simulink model "soc_dvbs2_fpga"  (R2025b)
settings: Solver=FixedStepDiscrete  StartTime=0.0  StopTime=0  RelTol=1e-3
InitFcn:
  | soc_dvbs2_init;
values from neighbouring files (symbols this model uses):
  Rsym = 4e6    (= 4000000)    [soc_dvbs2_init.m]
  soc_dvbs2_txPacketBits = [1 1 0 1 0 1 1 1 0 1 1 1 ... (2972 elements, 2972x1)]    [soc_dvbs2_txPacketBits.mat]
  syncWord = (dec2bin(hex2dec('AC')) - '0').'    [soc_dvbs2_init.m]
  txDataOut = txobj(frameBits(:))    [soc_dvbs2_init.m]
  txFiltCoeff = txobj.pTxFilterCoeff    [soc_dvbs2_init.m]
undefined symbols (not defined in the file or in its folder): Add, coefficientsLog, coefficientsSqrt1, coefficientsSqrt2, dataBits, designMultirateFIR, noisePow, NumBits1, NumBits2, seedsURNG1, seedsURNG2, Shift, Slope1, Slope2, soc_dvbs2_designFIRFilter, txDataOutS1, txDataOutS10, txDataOutS12, txDataOutS13, txDataOutS14, txDataOutS15, txDataOutS16, txDataOutS18, txDataOutS19, txDataOutS2, txDataOutS20, txDataOutS21, txDataOutS22, txDataOutS24, txDataOutS25, txDataOutS26, txDataOutS27, txDataOutS3, txDataOutS4, txDataOutS5, txDataOutS6, txDataOutS7, txDataOutS8, txDataOutS9
libraries: simulink x214, hdlsllib x211, dspsigops x22, dsphdlfiltering2 x8, dsphdlsigops2 x5, commseqgen3 x5, dsphdlmathfun2 x3, hwlogicconnlib x2, whdledac x2, commhdlcrc x2, whdlutilities x1, whdlmod x1
(part 1 of 12)
settings Model: DataDictionary=dvbs2hdlReceiverData.sldd  DataTypeOverride=Off  SimulationMode=accelerator  Creator=The MathWorks, Inc.  LastModifiedBy=The MathWorks, Inc.
settings SolverCC: PositivePriorityOrder=on  MaxZcPerStep=1.0
settings DataIOCC: ReturnWorkspaceOutputs=off
settings OptimizationCC: BlockReduction=off  ConditionallyExecuteInputs=off  DefaultParameterBehavior=Inlined  InheritOutputTypeSmallerThanSingle=on  EnhancedBackFolding=on  PassReuseOutputArgsAs=Individual arguments  ZeroExternalMemoryAtStartup=off  ZeroInternalMemoryAtStartup=off  MaxStackSize=64  OptimizeBlockOrder=speed  DifferentSizesBufferReuse=on  OptimizationCustomize=off  EfficientTunableParamExpr=on
settings DebuggingCC: ArtificialAlgebraicLoopMsg=error  SingleTaskRateTransMsg=error  ParameterTunabilityLossMsg=error  UnconnectedInputMsg=warning  UnconnectedOutputMsg=warning  UnconnectedLineMsg=warning  SubsystemReferenceDiagnosticForUnitTest=warning
settings HardwareCC: ProdBitPerPointer=32.0  ProdBitPerSizeT=32.0  ProdBitPerPtrDiffT=32.0  ProdLargestAtomicFloat=None  ProdIntDivRoundTo=Undefined  ProdEndianess=Unspecified  ProdWordSize=32.0  ProdHWDeviceType=ASIC/FPGA->ASIC/FPGA  TargetBitPerLong=64.0  TargetBitPerPointer=64.0  TargetBitPerSizeT=64.0  TargetBitPerPtrDiffT=64.0  TargetLongLongMode=on  TargetIntDivRoundTo=Zero  TargetEndianess=LittleEndian  TargetWordSize=64.0  TargetHWDeviceType=Custom Processor->MATLAB Host Computer  ProdEqTarget=off  HardwareBoardFeatureSet=SoCBlockset
settings ModelReferenceCC: EnableRefExpFcnMdlSchedulingChecks=on
settings RTWCC: SystemTargetFile=ert.tlc  HardwareBoard=Xilinx Zynq UltraScale+ RFSoC ZCU111 Evaluation Kit  TLCOptions="-aInlineSetEventsForThisBaseRateFcn=TLC_FALSE -aSuppressMultiTaskScheduler=TLC_FALSE  -aRateBasedStepFcn=0"  TemplateMakefile=ert_default_tmf  Toolchain=Linaro AArch64 Linux v6.3.1  GPUComputeCapability=3.5  DLArmComputeVersion=19.05  Description=Embedded Coder
settings CodeAppCC: ForceParamTrailComments=on  IgnoreCustomStorageClasses=off  OperatorAnnotations=on  SimulinkDataObjDesc=on  SFDataObjDesc=on  InsertBlockDesc=on

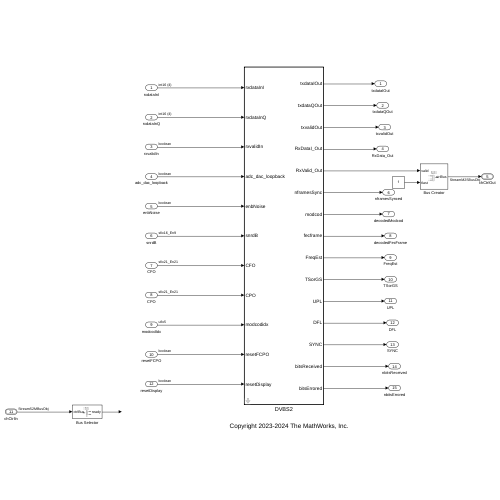
[thumbnail: Simulink's stored preview of the top-level diagram]
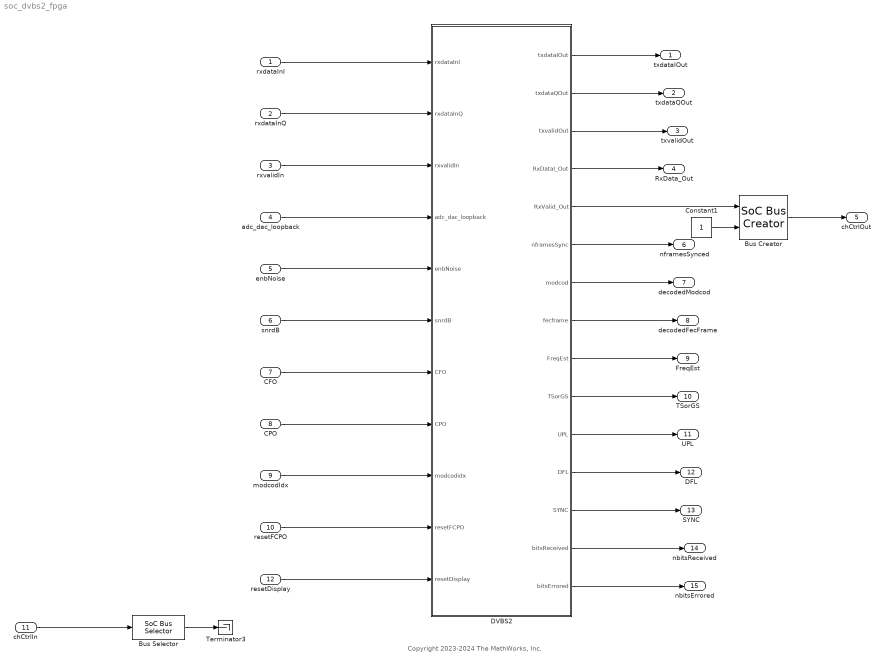
== system soc_dvbs2_fpga ==
  note: Copyright 2023-2024 The MathWorks, Inc.
  rxdataInI : Inport  OutDataTypeStr=int16  PortDimensions=4  LockScale=on
  rxdataInQ : Inport  Port=2  OutDataTypeStr=int16  PortDimensions=4  LockScale=on
  rxvalidIn : Inport  Port=3  OutDataTypeStr=boolean  LockScale=on
  adc_dac_loopback : Inport  Port=4  OutDataTypeStr=boolean  LockScale=on
  enbNoise : Inport  Port=5  OutDataTypeStr=boolean
  snrdB : Inport  Port=6  OutDataTypeStr=fixdt(1,16,9)
  CFO : Inport  Port=7  OutDataTypeStr=fixdt(1,21,21)
  CPO : Inport  Port=8  OutDataTypeStr=fixdt(1,21,21)
  modcodIdx : Inport  Port=9  OutDataTypeStr=fixdt(0,5,0)
  resetFCPO : Inport  Port=10  OutDataTypeStr=boolean
  chCtrlIn : Inport  Port=11  OutDataTypeStr=Bus: StreamS2MBusObj  BusOutputAsStruct=on
  resetDisplay : Inport  Port=12  OutDataTypeStr=boolean
  Bus Creator : hwlogicconnlib/SoC Bus Creator  Protocol=Data stream  ctrltype=Valid
  Bus Selector : hwlogicconnlib/SoC Bus Selector  Protocol=Data stream  ctrltype=Ready
  Constant1 : Constant  OutDataTypeStr=boolean  SampleTime=-1
  DVBS2 : Subsystem  TreatAsAtomicUnit=on
      mask init:
      | coe = designMultirateFIR(1,8); %#ok<NASGU> 
      | interp_coeff = designMultirateFIR(8,1,16); %#ok<NASGU> 
      | Simulink.suppressDiagnostic(gcb, 'SimulinkFixedPoint:util:fxpParameterPrecisionLoss');
  Terminator3 : Terminator
  txdataIOut : Outport
  txdataQOut : Outport  Port=2
  txvalidOut : Outport  Port=3
  RxData_Out : Outport  Port=4
  chCtrlOut : Outport  Port=5  OutDataTypeStr=Bus: StreamM2SBusObj  VectorParamsAs1DForOutWhenUnconnected=off  BusOutputAsStruct=on
  nframesSynced : Outport  Port=6
  decodedModcod : Outport  Port=7
  decodedFecFrame : Outport  Port=8
  FreqEst : Outport  Port=9
  TSorGS : Outport  Port=10
  UPL : Outport  Port=11
  DFL : Outport  Port=12
  SYNC : Outport  Port=13
  nbitsReceived : Outport  Port=14
  nbitsErrored : Outport  Port=15
  wires:
  rxdataInI/1 -> DVBS2/1(rxdataInI)
  rxdataInQ/1 -> DVBS2/2(rxdataInQ)
  rxvalidIn/1 -> DVBS2/3(rxvalidIn)
  adc_dac_loopback/1 -> DVBS2/4(adc_dac_loopback)
  snrdB/1 -> DVBS2/6(snrdB)
  CPO/1 -> DVBS2/8(CPO)
  modcodIdx/1 -> DVBS2/9(modcodidx)
  enbNoise/1 -> DVBS2/5(enbNoise)
  DVBS2/3(txvalidOut) -> txvalidOut/1
  DVBS2/6(nframesSync) -> nframesSynced/1
  DVBS2/7(modcod) -> decodedModcod/1
  DVBS2/8(fecframe) -> decodedFecFrame/1
  DVBS2/9(FreqEst) -> FreqEst/1
  resetFCPO/1 -> DVBS2/10(resetFCPO)
  DVBS2/4(RxDataI_Out) -> RxData_Out/1
  Bus Creator/1 -> chCtrlOut/1
  DVBS2/5(RxValid_Out) -> Bus Creator/1
  Constant1/1 -> Bus Creator/2
  chCtrlIn/1 -> Bus Selector/1
  Bus Selector/1 -> Terminator3/1
  CFO/1 -> DVBS2/7(CFO)
  DVBS2/1(txdataIOut) -> txdataIOut/1
  DVBS2/2(txdataQOut) -> txdataQOut/1
  DVBS2/11(UPL) -> UPL/1
  DVBS2/13(SYNC) -> SYNC/1
  DVBS2/10(TSorGS) -> TSorGS/1
  DVBS2/12(DFL) -> DFL/1
  DVBS2/14(bitsReceived) -> nbitsReceived/1
  DVBS2/15(bitsErrored) -> nbitsErrored/1
  resetDisplay/1 -> DVBS2/11(resetDisplay)

== system soc_dvbs2_fpga/DVBS2 ==
  rxdataInI : Inport
  rxdataInQ : Inport  Port=2
  rxvalidIn : Inport  Port=3
  adc_dac_loopback : Inport  Port=4
  enbNoise : Inport  Port=5
  snrdB : Inport  Port=6
  CFO : Inport  Port=7
  CPO : Inport  Port=8
  modcodidx : Inport  Port=9
  resetFCPO : Inport  Port=10
  resetDisplay : Inport  Port=11
  BER : Subsystem
  Bit Shift : hdlsllib/Logic and Bit Operations/Bit Shift  mode=Shift Left Logical  N=2
  Bit Shift1 : hdlsllib/Logic and Bit Operations/Bit Shift  mode=Shift Left Logical  N=2
  Concatention : Subsystem  TreatAsAtomicUnit=on
  DVBS2 TxRx : Subsystem
  Downsample{,1..6} (7 alike) : DownSample  N=8  RateOptions=Allow multirate processing
  Repeat{,1..2,4} (4 alike) : dspsigops/Repeat  FactorSource=Dialog parameter  N=32  Nmax=16  RateOptions=Allow multirate processing  ic=0  mode=Unused parameter value
  Upsample : dspsigops/Upsample  FactorSource=Dialog parameter  N=32  Nmax=16  phase=0  RateOptions=Allow multirate processing  ic=0  mode=Unused parameter value
  Upsample1 : dspsigops/Upsample  FactorSource=Dialog parameter  N=32  Nmax=16  phase=0  RateOptions=Allow multirate processing  ic=0  mode=Unused parameter value
  Vector Decimation : Subsystem
  Vector Interpolation : Subsystem
  txdataIOut : Outport
  txdataQOut : Outport  Port=2
  txvalidOut : Outport  Port=3
  RxDataI_Out : Outport  Port=4
  RxValid_Out : Outport  Port=5
  nframesSync : Outport  Port=6
  modcod : Outport  Port=7
  fecframe : Outport  Port=8
  FreqEst : Outport  Port=9
  TSorGS : Outport  Port=10
  UPL : Outport  Port=11
  DFL : Outport  Port=12
  SYNC : Outport  Port=13
  bitsReceived : Outport  Port=14
  bitsErrored : Outport  Port=15
  wires:
  adc_dac_loopback/1 -> Downsample/1
  CFO/1 -> Downsample3/1
  snrdB/1 -> Downsample2/1
  CPO/1 -> Downsample4/1
  resetFCPO/1 -> Downsample6/1
  modcodidx/1 -> Downsample5/1
  enbNoise/1 -> Downsample1/1
  DVBS2 TxRx/1(txDataI_Out) -> Vector Interpolation/1(dataI_in)
  DVBS2 TxRx/2(txDataQ_Out) -> Vector Interpolation/2(dataQ_in)
  DVBS2 TxRx/3(txValid_Out) -> Vector Interpolation/3(valid)
  Concatention/1(dataOut) -> RxDataI_Out/1
  Repeat/1 -> nframesSync/1
  Repeat1/1 -> modcod/1
  Repeat2/1 -> fecframe/1
  Repeat4/1 -> FreqEst/1
  Upsample/1 -> Concatention/1(dataIn)
  Upsample1/1 -> RxValid_Out/1
  Vector Decimation/1(dataIOut) -> DVBS2 TxRx/1(rxExtdataI_In)
  Vector Decimation/2(dataQOut) -> DVBS2 TxRx/2(rxExtdataQ_In)
  Vector Decimation/3(validOut) -> DVBS2 TxRx/3(rxExtValid_In)
  rxdataInI/1 -> Vector Decimation/1(dataI_in)
  rxvalidIn/1 -> Vector Decimation/3(validIn)
  Vector Interpolation/1(txIData) -> Bit Shift/1
  Vector Interpolation/2(txQData) -> Bit Shift1/1
  Vector Interpolation/3(txValid) -> txvalidOut/1
  rxdataInQ/1 -> Vector Decimation/2(dataQ_in)
  Bit Shift/1 -> txdataIOut/1
  Bit Shift1/1 -> txdataQOut/1
  DVBS2 TxRx/4(constlOut) -> Upsample/1
  DVBS2 TxRx/5(constlValid) -> Upsample1/1
  DVBS2 TxRx/6(nframesSync) -> Repeat/1
  DVBS2 TxRx/7(modcod) -> Repeat1/1
  DVBS2 TxRx/8(fecFrame) -> Repeat2/1
  DVBS2 TxRx/9(FreqEst) -> Repeat4/1
  DVBS2 TxRx/12(DFL) -> DFL/1
  DVBS2 TxRx/11(UPL) -> UPL/1
  DVBS2 TxRx/10(TsorGS) -> TSorGS/1
  DVBS2 TxRx/13(SYNC) -> SYNC/1
  DVBS2 TxRx/14(bitsOut) -> BER/1(userBits)
  DVBS2 TxRx/15(startOut) -> BER/2(srt)
  DVBS2 TxRx/16(endOut) -> BER/3(end)
  DVBS2 TxRx/17(validOut) -> BER/4(userBitsValid)
  DVBS2 TxRx/18(invalidPkt) -> BER/5(invalid)
  BER/1(bitCount) -> bitsReceived/1
  BER/2(bitErrors) -> bitsErrored/1
  resetDisplay/1 -> BER/6(resetcounter)
  Downsample/1 -> DVBS2 TxRx/4(adc_dac_loopback)
  Downsample1/1 -> DVBS2 TxRx/5(enNoise)
  Downsample2/1 -> DVBS2 TxRx/6(snrdB)
  Downsample3/1 -> DVBS2 TxRx/7(CFO)
  Downsample4/1 -> DVBS2 TxRx/8(CPO)
  Downsample5/1 -> DVBS2 TxRx/9(modcodidx)
  Downsample6/1 -> DVBS2 TxRx/10(rstFCPO)

== system soc_dvbs2_fpga/DVBS2/BER ==
  userBits : Inport
  srt : Inport  Port=2
  end : Inport  Port=3
  userBitsValid : Inport  Port=4
  invalid : Inport  Port=5
  resetcounter : Inport  Port=6
  Compare To Constant : simulink/Logic and Bit Operations/Compare To Constant  relop===  const=0  OutDataTypeStr=boolean
  Data Type Conversion1 : DataTypeConversion  OutDataTypeStr=boolean  SaturateOnIntegerOverflow=off  RndMeth=Floor
  Delay : Delay  DelayLength=1
  Delay1 : Delay  DelayLength=1
  Delay4 : Delay  DelayLength=1550
  Delay5 : Delay  DelayLength=1550
  Delay6 : Delay  DelayLength=1550
  HDL Counter : hdlsllib/Sources/HDL Counter  CountType=Free running  CountInit=0  CountStep=1  CountMax=25  CountFromType=Initial value  CountFrom=0  CountResetPort=on  CountLoadPort=off  CountEnbPort=on  CountDirPort=off  CountHitOutputPort=off  CountDataType=Unsigned  CountWordLen=32  CountFracLen=0  CountSampTime=1
  HDL Counter1 : hdlsllib/Sources/HDL Counter  CountType=Free running  CountInit=0  CountStep=1  CountMax=25  CountFromType=Initial value  CountFrom=0  CountResetPort=on  CountLoadPort=off  CountEnbPort=on  CountDirPort=off  CountHitOutputPort=off  CountDataType=Unsigned  CountWordLen=32  CountFracLen=0  CountSampTime=1
  Logical Operator : Logic  AllPortsSameDT=off  OutDataTypeStr=boolean
  Logical Operator1 : Logic  Operator=OR  AllPortsSameDT=off  OutDataTypeStr=boolean
  Logical Operator2 : Logic  Operator=NOT  AllPortsSameDT=off  OutDataTypeStr=boolean
  Logical Operator3 : Logic  AllPortsSameDT=off  OutDataTypeStr=boolean
  Relational Operator : RelationalOperator  Operator=~=  OutDataTypeStr=boolean  InputSameDT=off
  Send Payload Data : Subsystem  TreatAsAtomicUnit=on
  Unit Delay Enabled Synchronous : hdlsllib/Discrete/Unit Delay Enabled Synchronous  InitialCondition=0.0  SampleTime=-1
  Unit Delay Enabled Synchronous1 : hdlsllib/Discrete/Unit Delay Enabled Synchronous  InitialCondition=0.0  SampleTime=-1
  bitCount : Outport  VectorParamsAs1DForOutWhenUnconnected=off
  bitErrors : Outport  Port=2  VectorParamsAs1DForOutWhenUnconnected=off
  wires:
  Delay/1 -> Relational Operator/1
  Logical Operator3/1 -> Send Payload Data/2(nxtBit), HDL Counter1/2, Logical Operator/1
  Send Payload Data/1(dataIn) -> Data Type Conversion1/1
  Data Type Conversion1/1 -> Relational Operator/2
  Relational Operator/1 -> Logical Operator/2
  Logical Operator/1 -> HDL Counter/2
  HDL Counter1/1 -> Compare To Constant/1, bitCount/1
  HDL Counter/1 -> bitErrors/1
  srt/1 -> Delay6/1
  Compare To Constant/1 -> Logical Operator1/1
  Logical Operator1/1 -> HDL Counter/1
  resetcounter/1 -> Logical Operator1/2, HDL Counter1/1
  userBits/1 -> Delay5/1
  userBitsValid/1 -> Delay4/1
  invalid/1 -> Unit Delay Enabled Synchronous/1
  end/1 -> Unit Delay Enabled Synchronous/2
  Delay4/1 -> Delay1/1
  Delay5/1 -> Delay/1
  Delay6/1 -> Unit Delay Enabled Synchronous1/2, Send Payload Data/1(rst)
  Unit Delay Enabled Synchronous/1 -> Logical Operator2/1
  Logical Operator2/1 -> Unit Delay Enabled Synchronous1/1
  Delay1/1 -> Logical Operator3/2
  Unit Delay Enabled Synchronous1/1 -> Logical Operator3/1

== system soc_dvbs2_fpga/DVBS2/Concatention ==
  dataIn : Inport
  Bit Concat : hdlsllib/Logic and Bit Operations/Bit Concat  numInputs=2
  Complex to Real-Imag1 : ComplexToRealImag
  Data Type Conversion : DataTypeConversion  OutDataTypeStr=fixdt(1,16,12)  SaturateOnIntegerOverflow=off  RndMeth=Floor
  Data Type Conversion1 : DataTypeConversion  OutDataTypeStr=int16  ConvertRealWorld=Stored Integer (SI)  SaturateOnIntegerOverflow=off  RndMeth=Floor
  dataOut : Outport
  wires:
  Bit Concat/1 -> dataOut/1
  dataIn/1 -> Data Type Conversion/1
  Complex to Real-Imag1/1 -> Bit Concat/1
  Complex to Real-Imag1/2 -> Bit Concat/2
  Data Type Conversion/1 -> Data Type Conversion1/1
  Data Type Conversion1/1 -> Complex to Real-Imag1/1

== system soc_dvbs2_fpga/DVBS2/DVBS2 TxRx ==
  rxExtdataI_In : Inport
  rxExtdataQ_In : Inport  Port=2
  rxExtValid_In : Inport  Port=3
  adc_dac_loopback : Inport  Port=4
  enNoise : Inport  Port=5
  snrdB : Inport  Port=6
  CFO : Inport  Port=7
  CPO : Inport  Port=8
  modcodidx : Inport  Port=9
  rstFCPO : Inport  Port=10
  Bus Selector : BusSelector  OutputSignals=TSorGS,UPL,DFL,SYNC
  Channel : Subsystem
  Complex to Real-Imag : ComplexToRealImag
  DVB-S2 HDL Receiver : Subsystem
  Digital Automatic Gain Control : Subsystem  mask{desiredOutputPower=0.25, stepSize=(5e-4)}
      mask prompts: desiredOutputPower "Desired output power:"; stepSize "Adaptation step size:"
      mask init:
      | validateattributes(desiredOutputPower,{'double'},{'scalar','real','>=',0.125,'<=',2},'','desired output power');
      |    validateattributes(stepSize,{'double'},{'scalar','real','>=',0.5e-4,'<=',15e-4},'','step size');
      |    if desiredOutputPower > 1
      |        slopeAdj = 2^nextpow2(desiredOutputPower); %#ok<NASGU> 
      |    else
      |        slopeAdj = 1; %#ok<NASGU> 
      |    end
      mask DialogControl DescGroupVar Prompt: Digital Automatic Gain Control
      mask DialogControl DescTextVar Prompt: This block uses feedback loop based gain correction that adjusts adaptively to set the output signal level to reference level.
      mask Display:
      | dispstr1 = 'Digital AGC';
      | disp(dispstr1);
  Downsample7 : DownSample  N=4  RateOptions=Allow multirate processing
  LUT Based Tx : Subsystem
  Prepare Inputs : Subsystem
  Prepare Outputs : Subsystem
  Real-Imag to Complex : RealImagToComplex
  Switch : Switch  Criteria=u2 ~= 0  SaturateOnIntegerOverflow=off  InputSameDT=off
  Switch1 : Switch  Criteria=u2 ~= 0  SaturateOnIntegerOverflow=off  InputSameDT=off
  Terminator : Terminator
  Terminator1 : Terminator
  txDataI_Out : Outport
  txDataQ_Out : Outport  Port=2
  txValid_Out : Outport  Port=3
  constlOut : Outport  Port=4
  constlValid : Outport  Port=5
  nframesSync : Outport  Port=6
  modcod : Outport  Port=7
  fecFrame : Outport  Port=8
  FreqEst : Outport  Port=9
  TsorGS : Outport  Port=10
  UPL : Outport  Port=11
  DFL : Outport  Port=12
  SYNC : Outport  Port=13
  bitsOut : Outport  Port=14
  startOut : Outport  Port=15
  endOut : Outport  Port=16
  validOut : Outport  Port=17
  invalidPkt : Outport  Port=18
  wires:
  Switch/1 -> Digital Automatic Gain Control/1(dataIn)
  Switch1/1 -> Digital Automatic Gain Control/2(validIn)
  Digital Automatic Gain Control/1(dataOut) -> DVB-S2 HDL Receiver/1(dataIn)
  Digital Automatic Gain Control/2(validOut) -> DVB-S2 HDL Receiver/2(validIn)
  LUT Based Tx/2(txValidOut) -> Prepare Outputs/2(txvalid), Channel/2(txValidOut)
  adc_dac_loopback/1 -> Switch/2, Switch1/2
  CFO/1 -> Channel/5(CFO)
  snrdB/1 -> Channel/3(snrdB)
  CPO/1 -> Channel/6(CPO)
  rstFCPO/1 -> DVB-S2 HDL Receiver/3(rstFCPO)
  enNoise/1 -> Channel/4(enNoise)
  rxExtdataI_In/1 -> Real-Imag to Complex/1
  rxExtdataQ_In/1 -> Real-Imag to Complex/2
  Real-Imag to Complex/1 -> Prepare Inputs/1(rxData)
  rxExtValid_In/1 -> Prepare Inputs/2(rxValid)
  Prepare Inputs/2(rxValidOut) -> Switch1/1
  Complex to Real-Imag/1 -> txDataI_Out/1
  Complex to Real-Imag/2 -> txDataQ_Out/1
  Prepare Inputs/1(rxDataOut) -> Switch/1
  Channel/2(validOut) -> Switch1/3
  Channel/1(dataOut) -> Switch/3
  modcodidx/1 -> Downsample7/1
  Downsample7/1 -> LUT Based Tx/1(modcodidx)
  DVB-S2 HDL Receiver/1(syncSymb) -> constlOut/1
  DVB-S2 HDL Receiver/2(syncSymbValid) -> constlValid/1
  DVB-S2 HDL Receiver/3(numSynced) -> nframesSync/1
  DVB-S2 HDL Receiver/4(MODCOD) -> modcod/1
  DVB-S2 HDL Receiver/5(fecFrame) -> fecFrame/1
  DVB-S2 HDL Receiver/6(fineFreqEst) -> FreqEst/1
  DVB-S2 HDL Receiver/7(bitsOut) -> bitsOut/1
  DVB-S2 HDL Receiver/11(errorOut) -> Terminator/1
  DVB-S2 HDL Receiver/8(startOut) -> startOut/1
  DVB-S2 HDL Receiver/9(endOut) -> endOut/1
  DVB-S2 HDL Receiver/10(validOut) -> validOut/1
  DVB-S2 HDL Receiver/12(invalidPkt) -> invalidPkt/1
  DVB-S2 HDL Receiver/13(BBHeaderCRCInfo) -> Terminator1/1
  DVB-S2 HDL Receiver/14(BBheaderParams) -> Bus Selector/1
  Bus Selector/1 -> TsorGS/1  "<TSorGS>"
  Bus Selector/2 -> UPL/1  "<UPL>"
  Bus Selector/3 -> DFL/1  "<DFL>"
  Bus Selector/4 -> SYNC/1  "<SYNC>"
  LUT Based Tx/1(txDataOut) -> Channel/1(txDataOut), Prepare Outputs/1(txData)
  Prepare Outputs/2(txValidOut) -> txValid_Out/1
  Prepare Outputs/1(txDataOut) -> Complex to Real-Imag/1

== system soc_dvbs2_fpga/DVBS2/Vector Decimation ==
  dataI_in : Inport
  dataQ_in : Inport  Port=2
  validIn : Inport  Port=3  PortDimensions=1
  Bit Shift : hdlsllib/Logic and Bit Operations/Bit Shift  mode=Shift Left Logical  N=4
  Complex to Real-Imag : ComplexToRealImag
  Vector Decimation : Subsystem
  dataIOut : Outport
  dataQOut : Outport  Port=2
  validOut : Outport  Port=3
  wires:
  Complex to Real-Imag/2 -> dataQOut/1
  Complex to Real-Imag/1 -> dataIOut/1
  validIn/1 -> Vector Decimation/3(vin)
  Vector Decimation/2(vout) -> validOut/1
  dataQ_in/1 -> Vector Decimation/2(din_img)
  Vector Decimation/1(dout) -> Bit Shift/1
  dataI_in/1 -> Vector Decimation/1(din_real)
  Bit Shift/1 -> Complex to Real-Imag/1

== system soc_dvbs2_fpga/DVBS2/Vector Interpolation ==
  dataI_in : Inport
  dataQ_in : Inport  Port=2
  valid : Inport  Port=3
  Complex to Real-Imag : ComplexToRealImag
  Data Type Conversion3 : DataTypeConversion  OutDataTypeStr=int16  SaturateOnIntegerOverflow=off  RndMeth=Floor
  Data Type Conversion4 : DataTypeConversion  OutDataTypeStr=int16  SaturateOnIntegerOverflow=off  RndMeth=Floor
  Extract Bits1 : simulink/Logic and Bit Operations/Extract Bits  bitsToExtract=Range starting with most significant bit  numBits=12  bitIdxRange=[0 7]  outScalingMode=Treat bit field as an integer
  Extract Bits2 : simulink/Logic and Bit Operations/Extract Bits  bitsToExtract=Range starting with most significant bit  numBits=12  bitIdxRange=[0 7]  outScalingMode=Treat bit field as an integer
  FIR Interpolator : dsphdlfiltering2/FIR Interpolator  NumeratorSource=Property  Numerator=designMultirateFIR(4,1,16)  NumeratorPrototype=[]  FilterStructure=Direct form systolic  InterpolationFactor=4  NumCycles=1  OptimizeSymmCoeff=off  SimulateUsing=Code generation  roundingMode=Floor  overflowMode=off  CoefficientsDataTypeStr=Inherit: Same word length as input  OutputDataTypeStr=fixdt(1,16,0)  ResetInputPort=off  HDLGlobalReset=off
  Real-Imag to Complex : RealImagToComplex
  Terminator : Terminator
  txIData : Outport
  txQData : Outport  Port=2
  txValid : Outport  Port=3
  wires:
  Extract Bits2/1 -> Data Type Conversion4/1
  Extract Bits1/1 -> Data Type Conversion3/1
  FIR Interpolator/3 -> Terminator/1
  Complex to Real-Imag/2 -> txQData/1
  Complex to Real-Imag/1 -> txIData/1
  dataQ_in/1 -> Extract Bits2/1
  dataI_in/1 -> Extract Bits1/1
  Data Type Conversion4/1 -> Real-Imag to Complex/2
  Data Type Conversion3/1 -> Real-Imag to Complex/1
  FIR Interpolator/2 -> txValid/1
  valid/1 -> FIR Interpolator/2
  FIR Interpolator/1 -> Complex to Real-Imag/1
  Real-Imag to Complex/1 -> FIR Interpolator/1

== system soc_dvbs2_fpga/DVBS2/BER/Send Payload Data ==
  rst : Inport
  nxtBit : Inport  Port=2
  1-D Lookup Table : Lookup_n-D  NumberOfTableDimensions=1  LookupTableObject=''  BreakpointsSpecification=Even spacing  BreakpointsForDimension1=0:length(dataBits)-1  BreakpointsForDimension1FirstPoint=0  BreakpointsForDimension2FirstPoint=10  BreakpointsForDimension2Spacing=12  IndexSearchMethod=Evenly spaced points  Table=[syncWord;soc_dvbs2_txPacketBits]  TableDataTypeStr=int8  InterpMethod=Flat  DiagnosticForOutOfRangeInput=Error  InternalRulePriority=Speed  OutDataTypeStr=int8  RndMeth=Simplest
  HDL Counter : hdlsllib/Sources/HDL Counter  CountType=Count limited  CountInit=0  CountStep=1  CountMax=length([syncWord;soc_dvbs2_txPacketBits])-1  CountFromType=Initial value  CountFrom=0  CountResetPort=on  CountLoadPort=off  CountEnbPort=on  CountDirPort=off  CountHitOutputPort=off  CountDataType=Unsigned  CountWordLen=nextpow2(length([syncWord;soc_dvbs2_txPacketBits])-1)  CountFracLen=0  CountSampTime=1
  dataIn : Outport  InitialOutput=0  VectorParamsAs1DForOutWhenUnconnected=off
  wires:
  1-D Lookup Table/1 -> dataIn/1
  HDL Counter/1 -> 1-D Lookup Table/1
  rst/1 -> HDL Counter/1
  nxtBit/1 -> HDL Counter/2

== system soc_dvbs2_fpga/DVBS2/DVBS2 TxRx/Channel ==
  txDataOut : Inport
  txValidOut : Inport  Port=2
  snrdB : Inport  Port=3
  enNoise : Inport  Port=4
  CFO : Inport  Port=5
  CPO : Inport  Port=6
  AWGN Generator : Subsystem
      mask init:
      | Simulink.suppressDiagnostic(gcb, 'SimulinkFixedPoint:util:fxpParameterPrecisionLoss');
  Add : Sum  Inputs=+-  OutDataTypeStr=Inherit: Same as first input
  Constant : Constant  Value=complex(0)  OutDataTypeStr=Inherit: Inherit via back propagation  SampleTime=-1
  Data Type Conversion : DataTypeConversion  OutDataTypeStr=fixdt(1,21,0)  ConvertRealWorld=Stored Integer (SI)  SaturateOnIntegerOverflow=off  RndMeth=Floor
  Data Type Conversion1 : DataTypeConversion  OutDataTypeStr=fixdt(1,21,0)  ConvertRealWorld=Stored Integer (SI)  SaturateOnIntegerOverflow=off  RndMeth=Floor
  Delay : Delay  DelayLength=6
  NCO : dsphdlsigops2/NCO  PhaseIncrementSource=Input port  PhaseIncrement=100  PhaseOffsetSource=Input port  PhaseOffset=0  DitherSource=None  NumDitherBits=4  SamplesPerFrame=1  LUTCompress=off  ResetAction=off  Waveform=Complex exponential  PhasePort=off  SimulateUsing=Code generation  AccumulatorWL=21  PhaseQuantization=on  NumQuantizerAccumulatorBits=14  OutputDataType=Binary point scaling  OutputWL=16  OutputFL=14
  Product : Product  OutDataTypeStr=Inherit: Same as first input
  Switch2 : Switch  Criteria=u2 ~= 0  SaturateOnIntegerOverflow=off  InputSameDT=off
  dataOut : Outport
  validOut : Outport  Port=2
  wires:
  Switch2/1 -> Add/2
  enNoise/1 -> Switch2/2
  Constant/1 -> Switch2/3
  txDataOut/1 -> Add/1
  AWGN Generator/1(awgn) -> Switch2/1
  Add/1 -> Delay/1
  snrdB/1 -> AWGN Generator/1(snrdB)
  txValidOut/1 -> NCO/3
  NCO/2 -> validOut/1
  CFO/1 -> Data Type Conversion/1
  CPO/1 -> Data Type Conversion1/1
  NCO/1 -> Product/2
  Product/1 -> dataOut/1
  Delay/1 -> Product/1
  Data Type Conversion/1 -> NCO/1
  Data Type Conversion1/1 -> NCO/2

== system soc_dvbs2_fpga/DVBS2/DVBS2 TxRx/DVB-S2 HDL Receiver ==
  note: Use this port to enable the CCFO
      | for higer carrier offsets
  note: Use this port to enable the CCFO
      | for higer carrier offsets
  dataIn : Inport  SampleTime=1/(Rsym*4)
  validIn : Inport  Port=2  SampleTime=1/(Rsym*4)
  rstFCPO : Inport  Port=3  SampleTime=1/(Rsym*4)
  Bus Creator : BusCreator  Inputs=11
  Bus Selector : BusSelector  OutputSignals=NormalizedCoarseFrequencyEstimate,NormalizedFineFrequencyEstimate
  Bus Selector1 : BusSelector  OutputSignals=MODCOD,FECFrame
  Bus Selector2 : BusSelector  OutputSignals=NormalizedFrequencyEstimates
  Bus Selector3 : BusSelector  OutputSignals=start,valid
  Data Type Conversion : DataTypeConversion  OutDataTypeStr=fixdt(0,16,14)  SaturateOnIntegerOverflow=off  RndMeth=Floor
  Demod Deinterleave and FECDecode : Subsystem  mask{Rsym=Rsym, FECFrame=Short}
      mask prompts: Rsym "Symbol Rate:"; FECFrame "FEC Frame Type :"
      mask init:
      | switch FECFrame
      |     case 1
      |         set_param([gcb '/FEC Decoding/DVB-S2 BCH Decoder'],'FECFrameType','Normal');
      |         FECFrameConst = false;
      |     case 2
      |         set_param([gcb '/FEC Decoding/DVB-S2 BCH Decoder'],'FECFrameType','Short');
      |         FECFrameConst = true;
      | end
      mask TypeOptions FECFrame: Normal | Short
      mask Display: disp(['FEC Frame Type: ' newline get_param(gcb,'FECFrame')])
  HDL Counter : hdlsllib/Sources/HDL Counter  CountType=Free running  CountInit=0  CountStep=1  CountMax=25  CountFromType=Initial value  CountFrom=0  CountResetPort=off  CountLoadPort=off  CountEnbPort=on  CountDirPort=off  CountHitOutputPort=off  CountDataType=Unsigned  CountWordLen=32  CountFracLen=0  CountSampTime=1
  No HDL : Subsystem
  No HDL1 : Subsystem
  No HDL2 : Subsystem
  Repeat : dspsigops/Repeat  FactorSource=Dialog parameter  N=32  Nmax=16  RateOptions=Allow multirate processing  ic=0  mode=Unused parameter value
  Repeat1 : dspsigops/Repeat  FactorSource=Dialog parameter  N=32  Nmax=16  RateOptions=Allow multirate processing  ic=0  mode=Unused parameter value
  Repeat2 : dspsigops/Repeat  FactorSource=Dialog parameter  N=32  Nmax=16  RateOptions=Allow multirate processing  ic=0  mode=Unused parameter value
  Stream Recovery : Subsystem  mask{Rsym=Rsym}
      mask prompts: Rsym "Symbol rate :"
  Synchronizer and PL Header Decoder : Subsystem  mask{Rsym=Rsym, CFCV=off, FFCV=on, CPCV=on, FPCV=on, modcodToZero=on}
      mask prompts: Rsym "Symbol Rate :"; CFCV "Enable coarse frequency correction"; FFCV "Enable fine frequency correction"; CPCV "Enable coarse phase correction"; FPCV "Enable fine phase correction"; modcodToZero "Force MODCOD to 0 during initial synchronization"
      mask init:
      | config = dvbs2hdlRxParameters;
  Terminator : Terminator
  Upsample : dspsigops/Upsample  FactorSource=Dialog parameter  N=32  Nmax=16  phase=0  RateOptions=Allow multirate processing  ic=0  mode=Unused parameter value
  Upsample1 : dspsigops/Upsample  FactorSource=Dialog parameter  N=32  Nmax=16  phase=0  RateOptions=Allow multirate processing  ic=0  mode=Unused parameter value
  Upsample2 : dspsigops/Upsample  FactorSource=Dialog parameter  N=32  Nmax=16  phase=0  RateOptions=Allow multirate processing  ic=0  mode=Unused parameter value
  syncSymb : Outport
  syncSymbValid : Outport  Port=2
  numSynced : Outport  Port=3
  MODCOD : Outport  Port=4
  fecFrame : Outport  Port=5
  fineFreqEst : Outport  Port=6
  bitsOut : Outport  Port=7  VectorParamsAs1DForOutWhenUnconnected=off
  startOut : Outport  Port=8  VectorParamsAs1DForOutWhenUnconnected=off
  endOut : Outport  Port=9  VectorParamsAs1DForOutWhenUnconnected=off
  validOut : Outport  Port=10  VectorParamsAs1DForOutWhenUnconnected=off
  errorOut : Outport  Port=11  VectorParamsAs1DForOutWhenUnconnected=off
  invalidPkt : Outport  Port=12  VectorParamsAs1DForOutWhenUnconnected=off
  BBHeaderCRCInfo : Outport  Port=13  VectorParamsAs1DForOutWhenUnconnected=off
  BBheaderParams : Outport  Port=14  VectorParamsAs1DForOutWhenUnconnected=off
  wires:
  Synchronizer and PL Header Decoder/5(headerInfo) -> No HDL/5(headerinfo), Bus Selector1/1  "HeaderInformation"
  Synchronizer and PL Header Decoder/3(endOfPLSC) -> No HDL/3(endOfPLSc), HDL Counter/1, Upsample2/1  "EndOfPLSC"
  Synchronizer and PL Header Decoder/4(varOut) -> No HDL/4(varEst), Data Type Conversion/1  "VarianceEstimate"
  rstFCPO/1 -> Synchronizer and PL Header Decoder/3(rstFCPO)
  dataIn/1 -> Synchronizer and PL Header Decoder/1(dataIn)
  validIn/1 -> Synchronizer and PL Header Decoder/2(validIn)
  Bus Selector1/1 -> Repeat1/1, MODCOD/1  "<MODCOD>"
  Bus Selector1/2 -> Repeat2/1, fecFrame/1  "<FECFrame>"
  Data Type Conversion/1 -> Repeat/1
  Synchronizer and PL Header Decoder/6(diagBus) -> Bus Selector2/1, No HDL/6(diagbus)  "diagBusPLHeaderEx"
  HDL Counter/1 -> numSynced/1
  Synchronizer and PL Header Decoder/1(dataOut) -> No HDL/1(symbDemodIndata), syncSymb/1, Upsample/1  "SymbolDemodInDataOut"
  Synchronizer and PL Header Decoder/2(validOut) -> No HDL/2(symbDemodInValid), syncSymbValid/1, Upsample1/1  "SymbolDemodInValidOut"
  Demod Deinterleave and FECDecode/1(bitsOut) -> Stream Recovery/1(bitsIn)
  Demod Deinterleave and FECDecode/2(ctrl) -> Bus Selector3/1
  Bus Selector3/1 -> Stream Recovery/2(startIn)  "<start>"
  Bus Selector3/2 -> Stream Recovery/3(validIn)  "<valid>"
  Demod Deinterleave and FECDecode/3(status) -> No HDL1/1(u)
  Stream Recovery/3(endOut) -> endOut/1
  Stream Recovery/2(startOut) -> startOut/1
  Stream Recovery/4(validOut) -> validOut/1
  Stream Recovery/1(bitsOut) -> bitsOut/1
  Stream Recovery/5(errorOut) -> errorOut/1
  Stream Recovery/6(invalidPkt) -> invalidPkt/1
  Stream Recovery/7(headerCRCInfo) -> BBHeaderCRCInfo/1
  Stream Recovery/14(MIS_ISI) -> Bus Creator/7  "MIS_ISI"
  Stream Recovery/10(CCMorACM) -> Bus Creator/3  "CCMorACM"
  Stream Recovery/9(SISorMIS) -> Bus Creator/2  "SISorMIS"
  Stream Recovery/12(NPD) -> Bus Creator/5  "NPD"
  Bus Creator/1 -> BBheaderParams/1
  Stream Recovery/8(TSorGS) -> Bus Creator/1  "TSorGS"
  Stream Recovery/13(RO) -> Bus Creator/6  "RO"
  Stream Recovery/11(ISSYI) -> Bus Creator/4  "ISSYI"
  Stream Recovery/15(UPL) -> No HDL2/2(DFL), No HDL2/1(UPL), Bus Creator/8  "UPL"
  Stream Recovery/16(DFL) -> Bus Creator/9  "DFL"
  Stream Recovery/17(SYNC) -> No HDL2/3(SYNC), Bus Creator/10  "SYNC"
  Stream Recovery/18(SYNCD) -> No HDL2/4(SYNCD), Bus Creator/11
  Stream Recovery/19(frameSrt) -> No HDL2/5(frameStart)
  Stream Recovery/20(frameEnd) -> No HDL2/6(frameEnd)
  Upsample/1 -> Demod Deinterleave and FECDecode/1(dataIn)
  Upsample1/1 -> Demod Deinterleave and FECDecode/2(validIn)
  Upsample2/1 -> Demod Deinterleave and FECDecode/3(endOfPLSC)
  Repeat/1 -> Demod Deinterleave and FECDecode/4(nVarIn)
  Repeat1/1 -> Demod Deinterleave and FECDecode/5(MODCOD)
  Repeat2/1 -> Demod Deinterleave and FECDecode/6(FECFrame)
  Bus Selector/2 -> fineFreqEst/1  "<NormalizedFineFrequencyEstimate>"
  Bus Selector/1 -> Terminator/1  "<NormalizedCoarseFrequencyEstimate>"
  Bus Selector2/1 -> Bus Selector/1  "<NormalizedFrequencyEstimates>"

== system soc_dvbs2_fpga/DVBS2/DVBS2 TxRx/Digital Automatic Gain Control ==
  dataIn : Inport
  validIn : Inport  Port=2
  Data Type Propagation : simulink/Signal Attributes/Data Type Propagation  PropDataType=fixdt(1, 16)  IfRefDouble=double  IfRefSingle=single  IsSigned=IsSigned1 or IsSigned2  NumBitsBase=max([NumBits1 NumBits2])  NumBitsMult=1  NumBitsAdd=0  NumBitsAllowFinal=-1  PropScaling=2^-10  ValuesUsedBestPrec=[5 -7]  SlopeBase=min([Slope1 Slope2])  SlopeMult=slopeAdj  SlopeAdd=0  BiasBase=Bias1  BiasMult=1  BiasAdd=0
  Data Type Conversion : DataTypeConversion  SaturateOnIntegerOverflow=off  RndMeth=Floor
  Delay{1..9} (9 alike) : Delay
  Error Detector : Subsystem
  Loop Filter : Subsystem
  Product : Product
  dataOut : Outport
  validOut : Outport  Port=2
  wires:
  Data Type Conversion/1 -> Delay2/1, Data Type Propagation/3
  Product/1 -> Data Type Conversion/1
  Delay9/1 -> validOut/1
  Delay8/1 -> dataOut/1
  dataIn/1 -> Delay7/1
  validIn/1 -> Delay6/1
  Delay5/1 -> Delay3/1
  Delay3/1 -> Delay9/1
  Delay4/1 -> Product/1, Data Type Propagation/1, Data Type Propagation/2
  Delay1/1 -> Product/2
  Loop Filter/1(gain) -> Delay1/1
  Error Detector/1(err) -> Loop Filter/1(err)
  Delay6/1 -> Delay5/1
  Delay7/1 -> Delay4/1
  Delay2/1 -> Delay8/1, Error Detector/1(dataIn)

== system soc_dvbs2_fpga/DVBS2/DVBS2 TxRx/LUT Based Tx ==
  modcodidx : Inport
  Constant : Constant  Value=true  SampleTime=1/Rsym
  Data Type Conversion1 : DataTypeConversion  OutDataTypeStr=fixdt(1,18,15)  SaturateOnIntegerOverflow=off  RndMeth=Floor
  Delay : Delay
  Delay1 : Delay
  Discrete FIR Filter HDL Optimized : dsphdlfiltering2/Discrete FIR Filter  NumeratorSource=Property  Numerator=txFiltCoeff  NumeratorPrototype=[]  FilterStructure=Direct form systolic  SerializationOption=Minimum number of cycles between valid input samples  NumCycles=2  NumberOfMultipliers=2  SimulateUsing=Code generation  roundingMode=Floor  overflowMode=off  CoefficientsDataTypeStr=Inherit: Same word length as input  OutputDataTypeStr=Inherit: Same word length as input  ResetInputPort=off  HDLGlobalReset=off  CoeffMultiplier=Multiplier  UseMultForPow2Coeff=on  FrameInputSymmOptim=off
  Repeat : dspsigops/Repeat  FactorSource=Dialog parameter  N=4  Nmax=16  RateOptions=Allow multirate processing  ic=0  mode=Unused parameter value
  Subsystem1 : Subsystem
  Upsample : dspsigops/Upsample  FactorSource=Dialog parameter  N=4  Nmax=16  phase=0  RateOptions=Allow multirate processing  ic=0  mode=Unused parameter value
  txDataOut : Outport
  txValidOut : Outport  Port=2
  wires:
  Upsample/1 -> Discrete FIR Filter HDL Optimized/1
  Constant/1 -> Delay/1, Subsystem1/2(enb)
  Repeat/1 -> Discrete FIR Filter HDL Optimized/2
  Discrete FIR Filter HDL Optimized/2 -> txValidOut/1
  Discrete FIR Filter HDL Optimized/1 -> Data Type Conversion1/1
  Data Type Conversion1/1 -> txDataOut/1
  Subsystem1/1(Out1) -> Delay1/1
  modcodidx/1 -> Subsystem1/1(modcodidx)
  Delay/1 -> Repeat/1
  Delay1/1 -> Upsample/1

== system soc_dvbs2_fpga/DVBS2/DVBS2 TxRx/Prepare Inputs ==
  rxData : Inport
  rxValid : Inport  Port=2
  Data Type Conversion : DataTypeConversion  OutDataTypeStr=fixdt(1,16,14)  ConvertRealWorld=Stored Integer (SI)  SaturateOnIntegerOverflow=off  RndMeth=Floor
  Data Type Conversion1 : DataTypeConversion  OutDataTypeStr=fixdt(1,18,15)  ConvertRealWorld=Stored Integer (SI)  SaturateOnIntegerOverflow=off  RndMeth=Floor
  Delay{,1..3} (4 alike) : Delay
  Discrete FIR Filter HDL Optimized1 : dsphdlfiltering2/Discrete FIR Filter  NumeratorSource=Property  Numerator=soc_dvbs2_designFIRFilter(32,1.35,8-1.35)  NumeratorPrototype=[]  FilterStructure=Direct form systolic  SerializationOption=Minimum number of cycles between valid input samples  NumCycles=2  NumberOfMultipliers=2  SimulateUsing=Code generation  roundingMode=Floor  overflowMode=off  CoefficientsDataTypeStr=Inherit: Same word length as input  OutputDataTypeStr=Inherit: Same word length as input  ResetInputPort=off  HDLGlobalReset=off  CoeffMultiplier=Multiplier  UseMultForPow2Coeff=on  FrameInputSymmOptim=off
  Downsample1 : DownSample  N=8  RateOptions=Allow multirate processing
  Downsample2 : DownSample  N=8  RateOptions=Allow multirate processing
  Gain : Gain  Gain=2  ParamDataTypeStr=fixdt(0,3,0)  OutDataTypeStr=Inherit: Same as input
  rxDataOut : Outport
  rxValidOut : Outport  Port=2
  wires:
  Delay/1 -> Gain/1
  Delay3/1 -> rxValidOut/1
  Delay2/1 -> Data Type Conversion1/1
  Delay1/1 -> Delay3/1
  rxData/1 -> Data Type Conversion/1
  Discrete FIR Filter HDL Optimized1/1 -> Downsample2/1
  Data Type Conversion/1 -> Discrete FIR Filter HDL Optimized1/1
  Discrete FIR Filter HDL Optimized1/2 -> Downsample1/1
  rxValid/1 -> Discrete FIR Filter HDL Optimized1/2
  Downsample2/1 -> Delay/1
  Downsample1/1 -> Delay1/1
  Gain/1 -> Delay2/1
  Data Type Conversion1/1 -> rxDataOut/1

== system soc_dvbs2_fpga/DVBS2/DVBS2 TxRx/Prepare Outputs ==
  note: Gain
  txData : Inport
  txvalid : Inport  Port=2
  Data Type Conversion2 : DataTypeConversion  OutDataTypeStr=int16  ConvertRealWorld=Stored Integer (SI)  SaturateOnIntegerOverflow=off  RndMeth=Floor
  Data Type Conversion3 : DataTypeConversion  OutDataTypeStr=fixdt(1,16,13)  SaturateOnIntegerOverflow=off  RndMeth=Floor
  Delay{4..7} (4 alike) : Delay
  Discrete FIR Filter HDL Optimized : dsphdlfiltering2/Discrete FIR Filter  NumeratorSource=Property  Numerator=soc_dvbs2_designFIRFilter(32,1.35,8-1.35)  NumeratorPrototype=[]  FilterStructure=Direct form systolic  SerializationOption=Minimum number of cycles between valid input samples  NumCycles=2  NumberOfMultipliers=2  SimulateUsing=Code generation  roundingMode=Floor  overflowMode=off  CoefficientsDataTypeStr=Inherit: Same word length as input  OutputDataTypeStr=Inherit: Same word length as input  ResetInputPort=off  HDLGlobalReset=off  CoeffMultiplier=Multiplier  UseMultForPow2Coeff=on  FrameInputSymmOptim=off
  Gain : Gain  Gain=8  ParamDataTypeStr=fixdt(0,4,0)  OutDataTypeStr=Inherit: Same as input
  Repeat : dspsigops/Repeat  FactorSource=Dialog parameter  N=8  Nmax=16  RateOptions=Allow multirate processing  ic=0  mode=Unused parameter value
  Upsample : dspsigops/Upsample  FactorSource=Dialog parameter  N=8  Nmax=16  phase=0  RateOptions=Allow multirate processing  ic=0  mode=Unused parameter value
  txDataOut : Outport
  txValidOut : Outport  Port=2
  wires:
  Discrete FIR Filter HDL Optimized/2 -> Delay6/1
  Discrete FIR Filter HDL Optimized/1 -> Delay4/1
  Gain/1 -> Delay5/1
  Data Type Conversion2/1 -> txDataOut/1
  Delay6/1 -> Delay7/1
  Delay7/1 -> txValidOut/1
  txvalid/1 -> Repeat/1
  Delay5/1 -> Data Type Conversion3/1
  Delay4/1 -> Gain/1
  txData/1 -> Upsample/1
  Data Type Conversion3/1 -> Data Type Conversion2/1
  Upsample/1 -> Discrete FIR Filter HDL Optimized/1
  Repeat/1 -> Discrete FIR Filter HDL Optimized/2

== system soc_dvbs2_fpga/DVBS2/Vector Decimation/Vector Decimation ==
  din_real : Inport
  din_img : Inport  Port=2
  vin : Inport  Port=3
  FIR Decimation HDL Optimized : dsphdlfiltering2/FIR Decimator  NumeratorSource=Property  Numerator=designMultirateFIR(1,4)  NumeratorPrototype=[]  FilterStructure=Direct form systolic  DecimationFactor=4  NumCycles=1  OptimizeSymmCoeff=off  SimulateUsing=Code generation  roundingMode=Floor  overflowMode=off  CoefficientsDataTypeStr=Inherit: Same word length as input  OutputDataTypeStr=fixdt(1,16,0)  ResetInputPort=off  HDLGlobalReset=off
  Real-Imag to Complex : RealImagToComplex
  dout : Outport  VectorParamsAs1DForOutWhenUnconnected=off
  vout : Outport  Port=2  VectorParamsAs1DForOutWhenUnconnected=off
  wires:
  FIR Decimation HDL Optimized/2 -> vout/1
  FIR Decimation HDL Optimized/1 -> dout/1
  vin/1 -> FIR Decimation HDL Optimized/2  "vin"
  Real-Imag to Complex/1 -> FIR Decimation HDL Optimized/1  "in2"
  din_img/1 -> Real-Imag to Complex/2  "in2"
  din_real/1 -> Real-Imag to Complex/1  "in2"

== system soc_dvbs2_fpga/DVBS2/DVBS2 TxRx/Channel/AWGN Generator ==
  snrdB : Inport  OutDataTypeStr=fixdt(1,16,9)  PortDimensions=1
  Delay1 : Delay  DelayLength=46
  Gaussian Noise With Given Variance : Subsystem
  Unit Variance Gaussian Noise : Subsystem
  dB to Linear Scale Converter : Subsystem
  awgn : Outport
  wires:
  snrdB/1 -> dB to Linear Scale Converter/1(snrdB)
  dB to Linear Scale Converter/1(noiseVar) -> Delay1/1
  Gaussian Noise With Given Variance/1(awgn) -> awgn/1
  Unit Variance Gaussian Noise/1(x0) -> Gaussian Noise With Given Variance/2(x0)
  Unit Variance Gaussian Noise/2(x1) -> Gaussian Noise With Given Variance/3(x1)
  Delay1/1 -> Gaussian Noise With Given Variance/1(noiseVar)

== system soc_dvbs2_fpga/DVBS2/DVBS2 TxRx/DVB-S2 HDL Receiver/Demod Deinterleave and FECDecode ==
  dataIn : Inport
  validIn : Inport  Port=2
  endOfPLSC : Inport  Port=3  SampleTime=1/(Rsym*32)
  nVarIn : Inport  Port=4
  MODCOD : Inport  Port=5
  FECFrame : Inport  Port=6
  Bit Concat : hdlsllib/Logic and Bit Operations/Bit Concat  numInputs=3
  DVBS2 HDL Deinterleaver : Subsystem  mask{mode=Deinterleaver, Tsamp=-1}
      mask prompts: mode "Mode :"; Tsamp "Sample Time"
      mask init:
      | switch mode
      |     case 1
      |         isInterleave = true;
      |     case 2
      |         isInterleave = false;
      |     otherwise
      |         error(['Invalid mode of ' mode]);
      | end
      | clear mode;
      | 
      | ConfigRx.RAMCapacity = 64800*2;
      | ConfigRx.ShortFrameLen = 16200;
      | ConfigRx.NormalFrameLen = 64800;
      mask TypeOptions mode: Interleaver | Deinterleaver
      mask Display: disp(['DVB-S2' newline 'HDL ' newline get_param(gcb,'mode')]);
  Data Type Conversion3 : DataTypeConversion  OutDataTypeStr=fixdt(1,8,4)  RndMeth=Floor
  Discard Unsupported Frames : Subsystem
  FEC Decoding : Subsystem
      settings: PortSchema="{\"entries\":[{\"content\":{\"sides\":[{\"content\":{\"connectorIds\":[\"In1\",\"In2\",\"In3\",\"In4\",\"In5\",\"In6\"]},\"type\":\"ConnectorPlacement.EquallySpacedRectSide\",\"uuid\":\"6a443fd3-2d1e-40c1-9c9f-d881f8373ba8\"},{\"content\":{\"connectorIds\":[\"Out1\",\"Out2\"],\"side\":\"RIGHT\"},\"type\":\"ConnectorPlacement.EquallySpacedRectSide\",\"uuid\":\"24a8bd98-6fc9-425a-95a4-a47bfbdf0a1f\"},{\"content\":{\"connectorIds\":[\"Out3\",\"Out4\"],\"side\":\"TOP\"},\"type\":\"ConnectorPlacement.EquallySpacedRectSide\",\"uuid\":\"8128b80a-b64d-469a-9a66-2925dbcbb10e\"}]},\"type\":\"ConnectorPlacement.EquallySpacedConnector\",\"uuid\":\"09ed908b-afa2-464e-a11f-9f8d3d1de805\"}],\"packageUris\":[\"http://schema.mathworks.com/mf0/Connector/R2020b\"],\"version\":\"1.0\"}"
  Symbol Demodulaor : Subsystem
      settings: PortSchema="{\"entries\":[{\"content\":{\"sides\":[{\"content\":{\"connectorIds\":[\"In1\",\"In2\",\"In3\",\"In4\",\"In5\",\"In6\",\"In7\"]},\"type\":\"ConnectorPlacement.EquallySpacedRectSide\",\"uuid\":\"8b3c5109-5c74-420d-a46e-f57193e36c3f\"},{\"content\":{\"connectorIds\":[\"Out1\",\"Out2\",\"Out3\",\"Out4\",\"Out5\",\"Out6\"],\"side\":\"RIGHT\"},\"type\":\"ConnectorPlacement.EquallySpacedRectSide\",\"uuid\":\"51446419-baab-476f-a02a-12305fec0212\"},{\"content\":{\"connectorIds\":[\"Out7\"],\"side\":\"TOP\"},\"type\":\"ConnectorPlacement.EquallySpacedRectSide\",\"uuid\":\"140c14aa-0adf-4c27-bd8a-a3c09c030375\"}]},\"type\":\"ConnectorPlacement.EquallySpacedConnector\",\"uuid\":\"4418379d-926e-4518-a30f-4d8b39c8b080\"}],\"packageUris\":[\"http://schema.mathworks.com/mf0/Connector/R2020b\"],\"version\":\"1.0\"}"
  Terminator : Terminator
  bitsOut : Outport
  ctrl : Outport  Port=2
  status : Outport  Port=3
  wires:
  endOfPLSC/1 -> Discard Unsupported Frames/1(endOfPLSC)
  validIn/1 -> Discard Unsupported Frames/3(validIn)
  Discard Unsupported Frames/2(validOut) -> Symbol Demodulaor/2(validIn)
  MODCOD/1 -> Discard Unsupported Frames/5(MODCOD)
  nVarIn/1 -> Discard Unsupported Frames/4(nVarIn)
  FECFrame/1 -> Discard Unsupported Frames/6(FECFrame)
  dataIn/1 -> Discard Unsupported Frames/2(dataIn)
  Symbol Demodulaor/7(symbolIgnored) -> Bit Concat/1
  Bit Concat/1 -> status/1
  Data Type Conversion3/1 -> DVBS2 HDL Deinterleaver/1(dataIn)
  Discard Unsupported Frames/1(dataOut) -> Symbol Demodulaor/1(dataIn)
  Discard Unsupported Frames/3(nVarOut) -> Symbol Demodulaor/3(nVarIn)
  Discard Unsupported Frames/4(paramCapture) -> Symbol Demodulaor/4(paramCapture)
  Discard Unsupported Frames/5(modIdx) -> Symbol Demodulaor/5(modIdx)
  Discard Unsupported Frames/6(codIdx) -> Symbol Demodulaor/6(codIdx)
  Discard Unsupported Frames/7(FECFrameOut) -> Symbol Demodulaor/7(FECFrame)
  Symbol Demodulaor/1(softBitsOut) -> Data Type Conversion3/1
  Symbol Demodulaor/2(validOut) -> DVBS2 HDL Deinterleaver/2(validIn)
  Symbol Demodulaor/3(paramCaptureOut) -> DVBS2 HDL Deinterleaver/3(paramValid)
  Symbol Demodulaor/4(modIdxOut) -> DVBS2 HDL Deinterleaver/4(modIdxIn)
  Symbol Demodulaor/5(codIdxOut) -> DVBS2 HDL Deinterleaver/5(codIdxIn)
  Symbol Demodulaor/6(fecframeOut) -> DVBS2 HDL Deinterleaver/6(fecframeIn)
  DVBS2 HDL Deinterleaver/1(rd_dout) -> FEC Decoding/1(dataIn)
  DVBS2 HDL Deinterleaver/2(rd_startOut) -> FEC Decoding/2(startIn)
  DVBS2 HDL Deinterleaver/3(rd_endOut) -> FEC Decoding/3(endIn)
  DVBS2 HDL Deinterleaver/4(rd_validOut) -> FEC Decoding/4(validIn)
  DVBS2 HDL Deinterleaver/5(fecframe) -> FEC Decoding/5(FECFrame)
  DVBS2 HDL Deinterleaver/6(codIdx) -> FEC Decoding/6(codIdx)
  FEC Decoding/3(LDPCFrameIgnored) -> Bit Concat/2
  FEC Decoding/4(BCHFrameIgnored) -> Bit Concat/3
  FEC Decoding/1(bitsOut) -> bitsOut/1
  FEC Decoding/2(ctrl) -> ctrl/1
  DVBS2 HDL Deinterleaver/7(modIdx) -> Terminator/1

== system soc_dvbs2_fpga/DVBS2/DVBS2 TxRx/DVB-S2 HDL Receiver/No HDL ==
  symbDemodIndata : Inport
  symbDemodInValid : Inport  Port=2
  endOfPLSc : Inport  Port=3
  varEst : Inport  Port=4
  headerinfo : Inport  Port=5
  diagbus : Inport  Port=6
  Bus Selector1 : BusSelector  OutputSignals=MODCOD,FECFrame
  Bus Selector2 : BusSelector  OutputSignals=SymbolSyncedSymbols
  Bus Selector3 : BusSelector  OutputSignals=SymbolSyncedValidOut,SymbolSyncedDataOut
  Constellation1 : Subsystem
  Constellation2 : Subsystem
  Terminator : Terminator
  To Workspace : ToWorkspace  VariableName=simDataOut  SampleTime=-1
      settings: Save2DSignal=2-D array (concatenate along first dimension)
  To Workspace1 : ToWorkspace  VariableName=simEndOfPLSC  SampleTime=-1
      settings: Save2DSignal=2-D array (concatenate along first dimension)
  To Workspace2 : ToWorkspace  VariableName=simValidOut  SampleTime=-1
      settings: Save2DSignal=2-D array (concatenate along first dimension)
  To Workspace3 : ToWorkspace  VariableName=simMODCOD  SampleTime=-1
      settings: Save2DSignal=2-D array (concatenate along first dimension)
  To Workspace4 : ToWorkspace  VariableName=simFECFrame  SampleTime=-1
      settings: Save2DSignal=2-D array (concatenate along first dimension)
  wires:
  varEst/1 -> Terminator/1
  diagbus/1 -> Bus Selector2/1
  symbDemodIndata/1 -> Constellation2/1(symbDemodIndata), To Workspace/1
  Bus Selector3/1 -> Constellation1/Enable  "<SymbolSyncedValidOut>"
  Bus Selector3/2 -> Constellation1/1(symbSyncOut)  "<SymbolSyncedDataOut>"
  Bus Selector2/1 -> Bus Selector3/1  "<SymbolSyncedSymbols>"
  headerinfo/1 -> Bus Selector1/1
  Bus Selector1/2 -> To Workspace4/1  "<FECFrame>"
  Bus Selector1/1 -> To Workspace3/1  "<MODCOD>"
  symbDemodInValid/1 -> Constellation2/Enable, To Workspace2/1
  endOfPLSc/1 -> To Workspace1/1

== system soc_dvbs2_fpga/DVBS2/DVBS2 TxRx/DVB-S2 HDL Receiver/No HDL1 ==
  u : Inport
  Assertion : Assertion  AssertionFailFcn=Invalid Status seen in DVBS2 Symbol Demodulator
  Assertion1 : Assertion  AssertionFailFcn=Invalid Status seen in DVBS2 LDPC Decoder
  Assertion2 : Assertion  AssertionFailFcn=Invalid Status seen in DVBS2 BCH Decoder
  Data Type Conversion : DataTypeConversion  OutDataTypeStr=boolean  SaturateOnIntegerOverflow=off  RndMeth=Floor
  Data Type Conversion1 : DataTypeConversion  OutDataTypeStr=boolean  SaturateOnIntegerOverflow=off  RndMeth=Floor
  Data Type Conversion2 : DataTypeConversion  OutDataTypeStr=boolean  SaturateOnIntegerOverflow=off  RndMeth=Floor
  Extract Bits : simulink/Logic and Bit Operations/Extract Bits  bitsToExtract=Range of bits  numBits=8  bitIdxRange=0  outScalingMode=Treat bit field as an integer
  Extract Bits1 : simulink/Logic and Bit Operations/Extract Bits  bitsToExtract=Range of bits  numBits=8  bitIdxRange=1  outScalingMode=Treat bit field as an integer
  Extract Bits2 : simulink/Logic and Bit Operations/Extract Bits  bitsToExtract=Range of bits  numBits=8  bitIdxRange=2  outScalingMode=Treat bit field as an integer
  Logical Operator : Logic  Operator=NOT  Inputs=1  AllPortsSameDT=off  OutDataTypeStr=boolean
  Logical Operator1 : Logic  Operator=NOT  Inputs=1  AllPortsSameDT=off  OutDataTypeStr=boolean
  Logical Operator2 : Logic  Operator=NOT  Inputs=1  AllPortsSameDT=off  OutDataTypeStr=boolean
  wires:
  u/1 -> Extract Bits2/1, Extract Bits1/1, Extract Bits/1
  Data Type Conversion/1 -> Logical Operator/1
  Extract Bits2/1 -> Data Type Conversion/1
  Logical Operator/1 -> Assertion/1
  Extract Bits1/1 -> Data Type Conversion1/1
  Extract Bits/1 -> Data Type Conversion2/1
  Data Type Conversion1/1 -> Logical Operator1/1
  Data Type Conversion2/1 -> Logical Operator2/1
  Logical Operator2/1 -> Assertion2/1
  Logical Operator1/1 -> Assertion1/1
